simulink model "H1_z"  (R2020b)
settings: Solver=VariableStepAuto  StartTime=0.0  StopTime=10.0  RelTol=1e-3
settings Model: Creator=user  LastModifiedBy=user
settings DataIOCC: SaveOutput=off  SaveTime=off

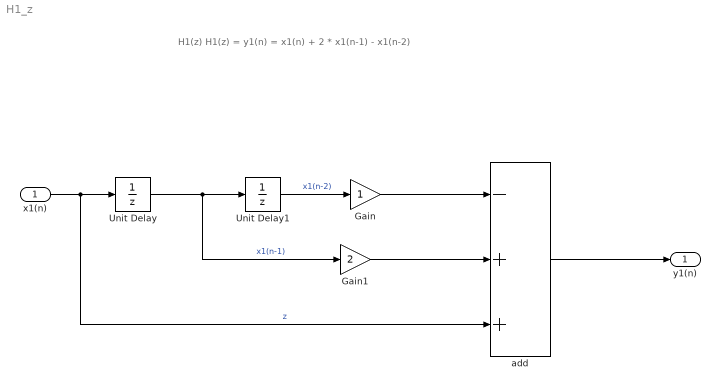
== system H1_z ==
  note: H1(z)
      |
      | H1(z) = y1(n) = x1(n) + 2 * x1(n-1) - x1(n-2)
  x1(n) : Inport  OutDataTypeStr=double  PortDimensions=1  SampleTime=0
  Gain : Gain
  Gain1 : Gain  Gain=2
  Unit Delay : UnitDelay  SampleTime=-1  HasFrameUpgradeWarning=on
  Unit Delay1 : UnitDelay  SampleTime=-1  HasFrameUpgradeWarning=on
  add : Sum  Inputs=-++
  y1(n) : Outport  OutDataTypeStr=double  PortDimensions=1  SampleTime=0
  wires:
  Gain/1 -> add/1
  add/1 -> y1(n)/1
  Gain1/1 -> add/2
  Unit Delay1/1 -> Gain/1  "x1(n-2)"
  Unit Delay/1 -> Unit Delay1/1, Gain1/1  "x1(n-1)"
  x1(n)/1 -> Unit Delay/1, add/3  "z"
